simulink model "Second_Order_Underdamped_System"  (R2024a)
settings: Solver=VariableStepAuto  StartTime=0.0  StopTime=20  RelTol=1e-3

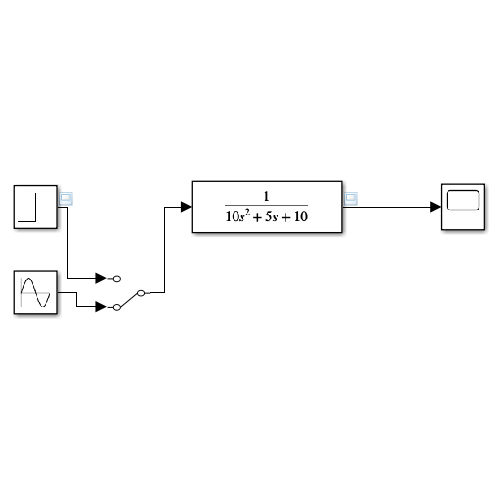
[thumbnail: Simulink's stored preview of the top-level diagram]
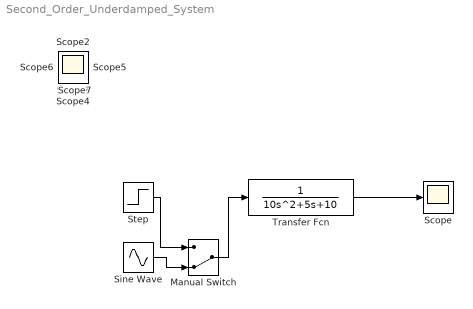
== system Second_Order_Underdamped_System ==
  Manual Switch : ManualSwitch  CurrentSetting=0
  Scope{,1..2,4..7} (7 alike) : Scope
  Sine Wave : Sin  SampleTime=0
  Step : Step  Time=0  Before=0.1  SampleTime=0
  Transfer Fcn : TransferFcn  Numerator=1  Denominator=[10 5 10]
  wires:
  Step/1 -> Manual Switch/1
  Transfer Fcn/1 -> Scope/1
  Sine Wave/1 -> Manual Switch/2
  Manual Switch/1 -> Transfer Fcn/1
